simulink model "regolatore_2"  (R2022b)
settings: Solver=VariableStepAuto  StartTime=0.0  StopTime=10.0  RelTol=1e-3
libraries: robotmobilelib x1
settings Model: Creator=thoma  LastModifiedBy=thoma

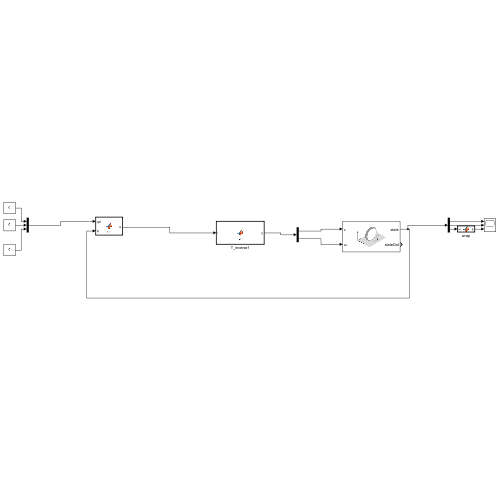
[thumbnail: Simulink's stored preview of the top-level diagram]
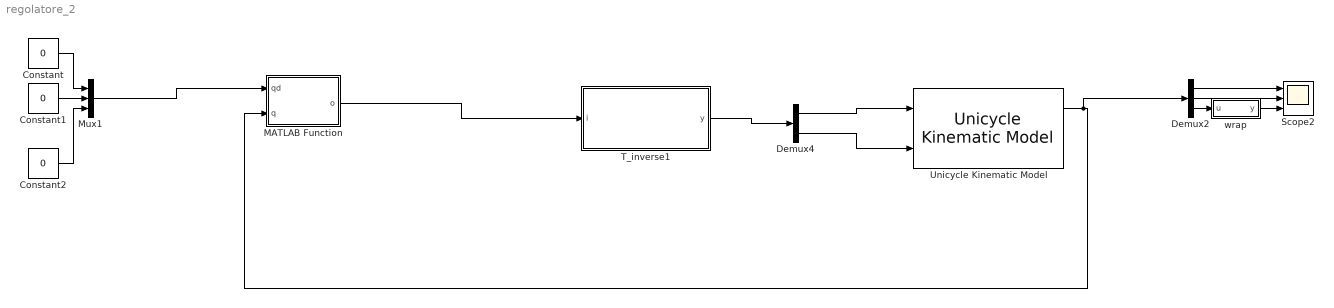
== system regolatore_2 ==
  Constant : Constant  Value=0
  Constant1 : Constant  Value=0
  Constant2 : Constant  Value=0
  Demux2 : Demux  Outputs=3
  Demux4 : Demux  Outputs=2
  MATLAB Function : MATLAB Function  TreatAsAtomicUnit=on
  Mux1 : Mux  Inputs=3
  Scope2 : Scope  NumInputPorts=3
  T_inverse1 : MATLAB Function  TreatAsAtomicUnit=on
  Unicycle Kinematic Model : robotmobilelib/Unicycle Kinematic Model  VehicleInputs=Vehicle Speed & Heading Angular Velocity  WheelRadius=2  WheelSpeedRange=[-Inf Inf]  InitialState=[1; 1; 1]  SimulateUsing=Interpreted execution
  wrap : MATLAB Function  TreatAsAtomicUnit=on
  wires:
  Demux4/2 -> Unicycle Kinematic Model/2
  Demux4/1 -> Unicycle Kinematic Model/1
  Constant/1 -> Mux1/1
  Unicycle Kinematic Model/1 -> Demux2/1, MATLAB Function/2(q)
  T_inverse1/1(y) -> Demux4/1
  Constant1/1 -> Mux1/2
  MATLAB Function/1(o) -> T_inverse1/1(i)
  Mux1/1 -> MATLAB Function/1(qd)
  Constant2/1 -> Mux1/3
  wrap/1(y) -> Scope2/3
  Demux2/1 -> Scope2/1
  Demux2/2 -> Scope2/2
  Demux2/3 -> wrap/1(u)

== matlab function regolatore_2/MATLAB Function ==
  data: qd input; o output; q input
function o = fcn(qd,q)
x=q(1);
y=q(2);
theta=q(3);
theta=mod(theta+pi,2*pi)-pi;
rho=sqrt(x^2+y^2);
gamma=atan2(y,x)+pi-theta;
delta=gamma+theta;
delta=mod(delta+pi,2*pi)-pi;
gamma=mod(gamma+pi,2*pi)-pi;
o = [rho;gamma;delta];

== matlab function regolatore_2/wrap ==
  data: u input; y output
function y = fcn(u)

y =mod(u+pi,2*pi)-pi;

== matlab function regolatore_2/T_inverse1 ==
  data: i input; y output
function y = fcn(i)
kv=10;
k1=3;
k2=10;
k3=1;
rho=i(1);
gamma=i(2);
delta=i(3);
v=k1*rho*cos(gamma);
w=k2*gamma+(k1* ((sin(gamma)*cos(gamma))/gamma) * (gamma+k3*delta));
y = [v;w];
